simulink model "z5234550RundongGuanPrimaryDT1_2020"  (R2020a)
settings: Solver=FixedStepDiscrete  StartTime=0.0  StopTime=1  FixedStep=Ts  RelTol=1e-3
InitFcn:
  | Ts = 1e-6;
  | Tcs = 100e-6;
  | Freq = 51.2;
undefined symbols (not defined in the file or in its folder): DiscIntNeverNeededParam
libraries: powerlib_meascontrol x2, z5234550RundongGuanLib_DT1_2020 x1, simulink x1
settings Model: Creator=Matthew Priestley  LastModifiedBy=Kevin
settings DataIOCC: SaveOutput=off  SignalLogging=off  DSMLogging=off  SaveTime=off  ReturnWorkspaceOutputs=off

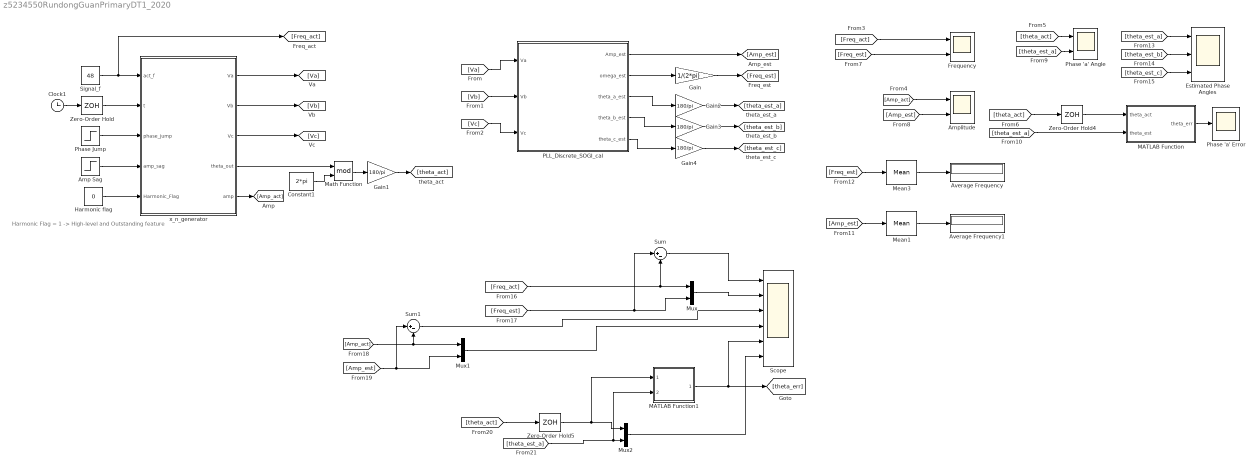
== system z5234550RundongGuanPrimaryDT1_2020 ==
  note: Harmonic Flag = 1 -> High-level and Outstanding feature
  Amp Sag : Step  Before=1  After=0.2  SampleTime=Ts
  Amplitude : Scope  NumInputPorts=2
  Average Frequency : Display
      settings: Decimation=5
  Average Frequency1 : Display
      settings: Decimation=5
  Clock1 : Clock
  Constant1 : Constant  Value=2*pi  SampleTime=Ts  LockScale=on
  Estimated Phase Angles : Scope  NumInputPorts=3
  Frequency : Scope  NumInputPorts=2
  Gain : Gain  Gain=1/(2*pi)
  Gain{1..4} (4 alike) : Gain  Gain=180/pi
  Harmonic flag : Constant  Value=0  SampleTime=Ts  LockScale=on
  MATLAB Function : MATLAB Function  TreatAsAtomicUnit=on
  MATLAB Function1 : MATLAB Function  TreatAsAtomicUnit=on
  Math Function : Math  Operator=mod  SignedPower=on  SaturateOnIntegerOverflow=on
  Mean1 : powerlib_meascontrol/Measurements/Mean  Freq=Freq  Vinit=0  Ts=Ts
  Mean3 : powerlib_meascontrol/Measurements/Mean  Freq=Freq  Vinit=0  Ts=Ts
  Mux : Mux  Inputs=2
  Mux1 : Mux  Inputs=2
  Mux2 : Mux  Inputs=2
  PLL_Discrete_SOGI_cal : Subsystem
  Phase 'a' Angle : Scope  NumInputPorts=2
  Phase 'a' Error : Scope
  Phase Jump : Step  Time=0.5  After=15  SampleTime=Ts
  Scope : Scope  NumInputPorts=6
  Signal_f : Constant  Value=48  SampleTime=Ts  LockScale=on
  Sum : Sum  Inputs=|+-
  Sum1 : Sum  Inputs=|+-
  Zero-Order Hold : ZeroOrderHold  SampleTime=Ts
  Zero-Order Hold4 : ZeroOrderHold  SampleTime=Tcs
  Zero-Order Hold5 : ZeroOrderHold  SampleTime=-1
  x_n_generator : MATLAB Function  TreatAsAtomicUnit=on
  wires:
  x_n_generator/4(theta_out) -> Math Function/1
  Zero-Order Hold/1 -> x_n_generator/2(t)
  x_n_generator/5(amp) -> [Amp_act]
  Phase Jump/1 -> x_n_generator/3(phase_jump)
  Amp Sag/1 -> x_n_generator/4(amp_sag)
  Clock1/1 -> Zero-Order Hold/1
  Math Function/1 -> Gain1/1
  Constant1/1 -> Math Function/2
  x_n_generator/2(Vb) -> [Vb]
  x_n_generator/1(Va) -> [Va]
  x_n_generator/3(Vc) -> [Vc]
  Harmonic flag/1 -> x_n_generator/5(Harmonic_Flag)
  [Freq_act] -> Frequency/1
  [Amp_act] -> Amplitude/1
  [theta_act] -> Phase 'a' Angle/1
  [theta_act] -> Zero-Order Hold4/1
  [Freq_est] -> Frequency/2
  [Amp_est] -> Amplitude/2
  [theta_est_a] -> Phase 'a' Angle/2
  MATLAB Function/1(theta_err) -> Phase 'a' Error/1
  [theta_est_a] -> MATLAB Function/2(theta_est)
  [Freq_est] -> Mean3/1
  Mean3/1 -> Average Frequency/1
  Gain1/1 -> [theta_act]
  [theta_est_a] -> Estimated Phase Angles/1
  [theta_est_b] -> Estimated Phase Angles/2
  [theta_est_c] -> Estimated Phase Angles/3
  Mux/1 -> Scope/2
  [Freq_act] -> Mux/1, Sum/2
  [Freq_est] -> Mux/2, Sum/1
  [Amp_act] -> Sum1/2, Mux1/1
  [Amp_est] -> Sum1/1, Mux1/2
  Mux1/1 -> Scope/4
  [theta_est_a] -> MATLAB Function1/2(theta_est), Mux2/2
  Mux2/1 -> Scope/6
  Zero-Order Hold4/1 -> MATLAB Function/1(theta_act)
  [theta_act] -> Zero-Order Hold5/1
  Zero-Order Hold5/1 -> Mux2/1, MATLAB Function1/1(theta_act)
  Gain/1 -> [Freq_est]
  Gain2/1 -> [theta_est_a]
  Gain3/1 -> [theta_est_b]
  Gain4/1 -> [theta_est_c]
  Sum/1 -> Scope/1
  Sum1/1 -> Scope/3
  MATLAB Function1/1(theta_err) -> [theta_err], Scope/5
  [Va] -> PLL_Discrete_SOGI_cal/1(Va)
  [Vb] -> PLL_Discrete_SOGI_cal/2(Vb)
  [Vc] -> PLL_Discrete_SOGI_cal/3(Vc)
  PLL_Discrete_SOGI_cal/2(omega_est) -> Gain/1
  PLL_Discrete_SOGI_cal/3(theta_a_est) -> Gain2/1
  PLL_Discrete_SOGI_cal/4(theta_b_est) -> Gain3/1
  PLL_Discrete_SOGI_cal/5(theta_c_est) -> Gain4/1
  PLL_Discrete_SOGI_cal/1(Amp_est) -> [Amp_est]
  Signal_f/1 -> [Freq_act], x_n_generator/1(act_f)
  Mean1/1 -> Average Frequency1/1
  [Amp_est] -> Mean1/1

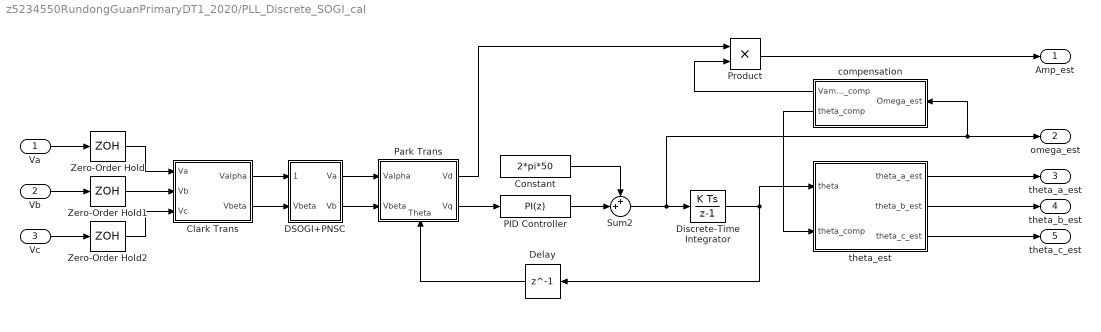
== system z5234550RundongGuanPrimaryDT1_2020/PLL_Discrete_SOGI_cal ==
  Va : Inport
  Vb : Inport  Port=2
  Vc : Inport  Port=3
  Clark Trans : Subsystem
  Constant : Constant  Value=2*pi*50  SampleTime=Tcs
  DSOGI+PNSC : Subsystem
  Delay : Delay  DelayLength=1  SampleTime=Tcs
  Discrete-Time Integrator : DiscreteIntegrator  SampleTime=Tcs  ICPrevOutput=DiscIntNeverNeededParam  ICPrevScaledInput=DiscIntNeverNeededParam
  PID Controller : simulink/Continuous/PID Controller  Controller=PI  Form=Parallel  TimeDomain=Discrete-time  UseExternalTs=off  SampleTime=Tcs  IntegratorMethod=Forward Euler  FilterMethod=Forward Euler  ControllerParametersSource=internal  P=4  I=100  D=0  UseFilter=on  N=100  TunerSelectOption=Transfer Function Based (PID Tuner App)  InitialConditionSource=internal  InitialConditionForIntegrator=0  InitialConditionForFilter=0  DifferentiatorICPrevScaledInput=0  ExternalReset=none  TrackingMode=off  Kt=1  LimitOutput=off  UpperSaturationLimit=inf  LowerSaturationLimit=-inf  LinearizeAsGain=on  AntiWindupMode=none  Kb=1  POutMin=[]  POutMax=[]  IOutMin=[]  IOutMax=[]  DOutMin=[]  DOutMax=[]  NOutMin=[]  NOutMax=[]  SumOutMin=[]  SumOutMax=[]  SaturationOutMin=[]  SaturationOutMax=[]  PParamMin=[]  PParamMax=[]  IParamMin=[]  IParamMax=[]  DParamMin=[]  DParamMax=[]  NParamMin=[]  NParamMax=[]  KbParamMin=[]  KbParamMax=[]  KtParamMin=[]  KtParamMax=[]  KbOutMin=[]  KbOutMax=[]  KtOutMin=[]  KtOutMax=[]  IntegratorOutMin=[]  IntegratorOutMax=[]  FilterOutMin=[]  FilterOutMax=[]  SumI1OutMin=[]  SumI1OutMax=[]  SumI2OutMin=[]  SumI2OutMax=[]  SumI3OutMin=[]  SumI3OutMax=[]  SumI4OutMin=[]  SumI4OutMax=[]  SumDOutMin=[]  SumDOutMax=[]  DifferentiatorOutMin=[]  DifferentiatorOutMax=[]  FilterDiffOutCoefMin=[]  FilterDiffOutCoefMax=[]  ReciprocalOutMin=[]  ReciprocalOutMax=[]  SumDenOutMin=[]  SumDenOutMax=[]  SumNumOutMin=[]  SumNumOutMax=[]  DivideOutMin=[]  DivideOutMax=[]  UdiffTsProdOutMin=[]  UdiffTsProdOutMax=[]  NTsProdOutMin=[]  NTsProdOutMax=[]  UintegralTsProdOutMin=[]  UintegralTsProdOutMax=[]  UngainTsProdOutMin=[]  UngainTsProdOutMax=[]  IntegratorContinuousStateAttributes=''  IntegratorStateMustResolveToSignalObject=off  IntegratorRTWStateStorageClass=Auto  FilterContinuousStateAttributes=''  FilterStateMustResolveToSignalObject=off  FilterRTWStateStorageClass=Auto  ParallelPVariant=InternalParameters  IdealPVariant=Disabled  IVariant=InternalParameters  DVariant=Disabled  IntegratorVariant=Discrete  SatVariant=Disabled  AWVariant=Passthrough  PCopyVariant=Disabled  TRVariant=Disabled  FdbkBlocksVariant=Forward  IdealPFdbkVariant=Disabled  SatFdbkVariant=Disabled  DerivativeFilterVariant=Disabled  NVariant=Disabled  NCopyVariant=Disabled_SignalSpec  FilterICVariant=Disabled  IntegratorICVariant=InternalICs  ExternalResetVariant=Disabled  TRSumVariant=Passthrough  SumFdbkVariant=Disabled  SumVariant=Sum_PI  TsampFilterVariant=InternalTs  TsampNgainVariant=Passthrough  TsampIntegralVariant=Passthrough
  Park Trans : Subsystem
      settings: PortSchema="{\"entries\":[{\"content\":{\"sides\":[{\"content\":{\"connectorIds\":[\"In1\",\"In2\"]},\"type\":\"ConnectorPlacement.EquallySpacedRectSide\",\"uuid\":\"d7ee73cc-3741-4077-b32c-689f2c701f83\"},{\"content\":{\"connectorIds\":[\"Out1\",\"Out2\"],\"side\":\"RIGHT\"},\"type\":\"ConnectorPlacement.EquallySpacedRectSide\",\"uuid\":\"fa84044a-ecd8-49d8-a4b2-ae549d89fe8f\"},{\"content\":{\"connectorIds\":[],\"side\":\"TOP\"},\"type\":\"ConnectorPlacement.EquallySpacedRectSide\",\"uuid\":\"692e7773-1833-4597-a5fd-7846ecf4550e\"},{\"content\":{\"connectorIds\":[\"In3\"],\"side\":\"BOTTOM\"},\"type\":\"ConnectorPlacement.EquallySpacedRectSide\",\"uuid\":\"73d654b9-9f56-4244-9824-eb13bf44a38f\"}]},\"type\":\"ConnectorPlacement.EquallySpacedConnector\",\"uuid\":\"4e0b4972-389e-416e-b0d9-9fdc8ba0f1f7\"}],\"packageUris\":[\"http://schema.mathworks.com/mf0/Connector/19700101\"],\"version\":\"1.0\"}"
  Product : Product
  Sum2 : Sum  Inputs=++|
  Zero-Order Hold : ZeroOrderHold  SampleTime=Tcs
  Zero-Order Hold1 : ZeroOrderHold  SampleTime=Tcs
  Zero-Order Hold2 : ZeroOrderHold  SampleTime=Tcs
  compensation : Subsystem
      settings: PortSchema="{\"entries\":[{\"content\":{\"sides\":[{\"content\":{\"connectorIds\":[\"Out1\",\"Out2\"]},\"type\":\"ConnectorPlacement.EquallySpacedRectSide\",\"uuid\":\"1da655cf-4ef1-485d-9c9d-29e08b49196c\"},{\"content\":{\"connectorIds\":[\"In1\"],\"side\":\"RIGHT\"},\"type\":\"ConnectorPlacement.EquallySpacedRectSide\",\"uuid\":\"274b50d4-d2b9-4d73-9fa7-29da8dc32335\"},{\"content\":{\"connectorIds\":[],\"side\":\"TOP\"},\"type\":\"ConnectorPlacement.EquallySpacedRectSide\",\"uuid\":\"51928977-61f6-4419-af9c-6bbf4ccbe560\"}]},\"type\":\"ConnectorPlacement.EquallySpacedConnector\",\"uuid\":\"bbbb2fbe-31dd-41e3-8294-b416b392d210\"}],\"packageUris\":[\"http://schema.mathworks.com/mf0/Connector/19700101\"],\"version\":\"1.0\"}"
  theta_est : Subsystem
  Amp_est : Outport
  omega_est : Outport  Port=2
  theta_a_est : Outport  Port=3
  theta_b_est : Outport  Port=4
  theta_c_est : Outport  Port=5
  wires:
  compensation/2(theta_comp) -> theta_est/2(theta_comp)
  Park Trans/1(Vd) -> Product/1
  compensation/1(Vamp_comp) -> Product/2
  Product/1 -> Amp_est/1
  Sum2/1 -> Discrete-Time Integrator/1, omega_est/1, compensation/1(Omega_est)
  Zero-Order Hold1/1 -> Clark Trans/2(Vb)
  Vc/1 -> Zero-Order Hold2/1
  Vb/1 -> Zero-Order Hold1/1
  Zero-Order Hold2/1 -> Clark Trans/3(Vc)
  Zero-Order Hold/1 -> Clark Trans/1(Va)
  Va/1 -> Zero-Order Hold/1
  theta_est/1(theta_a_est) -> theta_a_est/1
  theta_est/2(theta_b_est) -> theta_b_est/1
  theta_est/3(theta_c_est) -> theta_c_est/1
  Park Trans/2(Vq) -> PID Controller/1
  Clark Trans/1(Valpha) -> DSOGI+PNSC/1(Valpha)
  Clark Trans/2(Vbeta) -> DSOGI+PNSC/2(Vbeta)
  DSOGI+PNSC/1(Va) -> Park Trans/1(Valpha)
  DSOGI+PNSC/2(Vb) -> Park Trans/2(Vbeta)
  Delay/1 -> Park Trans/3(Theta)
  PID Controller/1 -> Sum2/2
  Constant/1 -> Sum2/1
  Discrete-Time Integrator/1 -> theta_est/1(theta), Delay/1

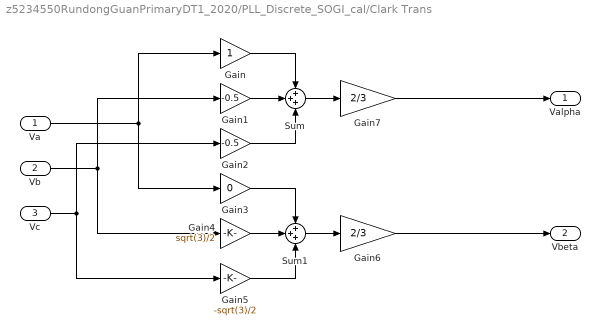
== system z5234550RundongGuanPrimaryDT1_2020/PLL_Discrete_SOGI_cal/Clark Trans ==
  Va : Inport
  Vb : Inport  Port=2
  Vc : Inport  Port=3
  Gain : Gain
  Gain1 : Gain  Gain=-0.5
  Gain2 : Gain  Gain=-0.5
  Gain3 : Gain  Gain=0
  Gain4 : Gain  Gain=sqrt(3)/2
  Gain5 : Gain  Gain=-sqrt(3)/2
  Gain6 : Gain  Gain=2/3
  Gain7 : Gain  Gain=2/3
  Sum : Sum  Inputs=+++
  Sum1 : Sum  Inputs=+++
  Valpha : Outport
  Vbeta : Outport  Port=2
  wires:
  Gain2/1 -> Sum/3
  Va/1 -> Gain3/1, Gain/1
  Vc/1 -> Gain5/1, Gain2/1
  Vb/1 -> Gain4/1, Gain1/1
  Gain/1 -> Sum/1
  Gain3/1 -> Sum1/1
  Gain1/1 -> Sum/2
  Gain5/1 -> Sum1/3
  Gain4/1 -> Sum1/2
  Sum/1 -> Gain7/1
  Sum1/1 -> Gain6/1
  Gain7/1 -> Valpha/1
  Gain6/1 -> Vbeta/1

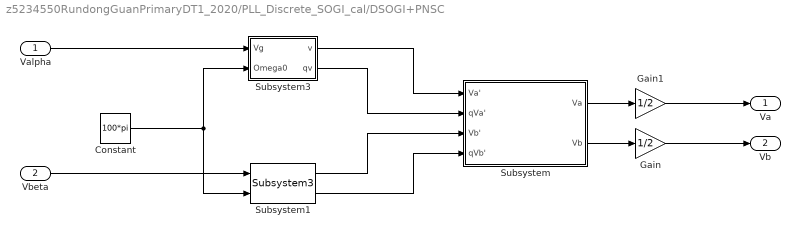
== system z5234550RundongGuanPrimaryDT1_2020/PLL_Discrete_SOGI_cal/DSOGI+PNSC ==
  Valpha : Inport
  Vbeta : Inport  Port=2
  Constant : Constant  Value=100*pi
  Gain : Gain  Gain=1/2
  Gain1 : Gain  Gain=1/2
  Subsystem : Subsystem
  Subsystem1 : z5234550RundongGuanLib_DT1_2020/PLL_Discrete_SOGI/DSOGI+PNSC/Subsystem3  SystemSampleTime=-1  Latency=0  AutoFrameSizeCalculation=off
      link override Gain: Gain=0.75
  Subsystem3 : Subsystem
  Va : Outport
  Vb : Outport  Port=2
  wires:
  Constant/1 -> Subsystem1/2, Subsystem3/2(Omega0)
  Subsystem3/1(v) -> Subsystem/1(Va')
  Subsystem3/2(qv) -> Subsystem/2(qVa')
  Subsystem/1(Va) -> Gain1/1
  Subsystem/2(Vb) -> Gain/1
  Valpha/1 -> Subsystem3/1(Vg)
  Vbeta/1 -> Subsystem1/1
  Subsystem1/1 -> Subsystem/3(Vb')
  Subsystem1/2 -> Subsystem/4(qVb')
  Gain1/1 -> Va/1
  Gain/1 -> Vb/1

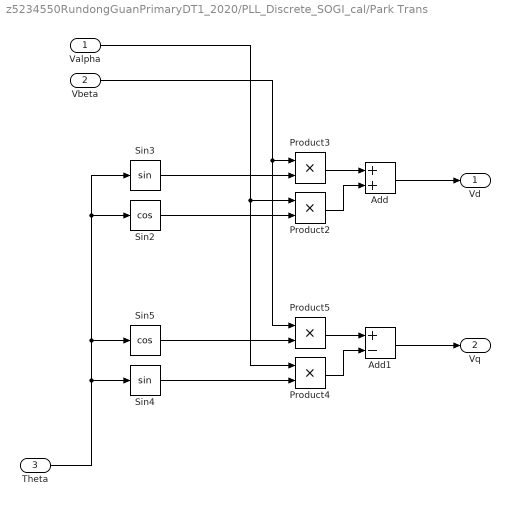
== system z5234550RundongGuanPrimaryDT1_2020/PLL_Discrete_SOGI_cal/Park Trans ==
  Valpha : Inport
  Vbeta : Inport  Port=2
  Theta : Inport  Port=3
  Add : Sum
  Add1 : Sum  Inputs=+-
  Product{2..5} (4 alike) : Product
  Sin2 : Trigonometry  Operator=cos
  Sin3 : Trigonometry
  Sin4 : Trigonometry
  Sin5 : Trigonometry  Operator=cos
  Vd : Outport
  Vq : Outport  Port=2
  wires:
  Vbeta/1 -> Product5/1, Product3/1
  Theta/1 -> Sin4/1, Sin5/1, Sin2/1, Sin3/1
  Sin5/1 -> Product5/2
  Valpha/1 -> Product2/1, Product4/1
  Product4/1 -> Add1/2
  Product2/1 -> Add/2
  Sin2/1 -> Product2/2
  Add/1 -> Vd/1
  Sin3/1 -> Product3/2
  Product3/1 -> Add/1
  Add1/1 -> Vq/1
  Sin4/1 -> Product4/2
  Product5/1 -> Add1/1

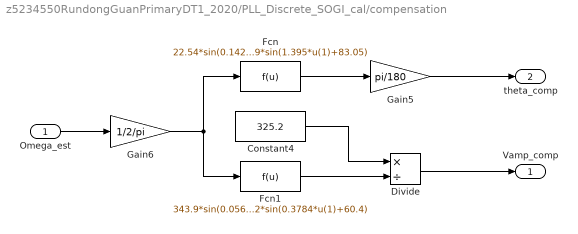
== system z5234550RundongGuanPrimaryDT1_2020/PLL_Discrete_SOGI_cal/compensation ==
  Omega_est : Inport
  Constant4 : Constant  Value=325.2
  Divide : Product  Inputs=*/
  Fcn : Fcn  Expr=22.54*sin(0.1425*u(1)+68.25)+0.07009*sin(1.395*u(1)+83.05)
  Fcn1 : Fcn  Expr=343.9*sin(0.05621*u(1)+36.6)+1.732*sin(0.3784*u(1)+60.4)
  Gain5 : Gain  Gain=pi/180
  Gain6 : Gain  Gain=1/2/pi
  Vamp_comp : Outport
  theta_comp : Outport  Port=2
  wires:
  Gain6/1 -> Fcn/1, Fcn1/1
  Omega_est/1 -> Gain6/1
  Divide/1 -> Vamp_comp/1
  Gain5/1 -> theta_comp/1
  Fcn/1 -> Gain5/1
  Constant4/1 -> Divide/1
  Fcn1/1 -> Divide/2

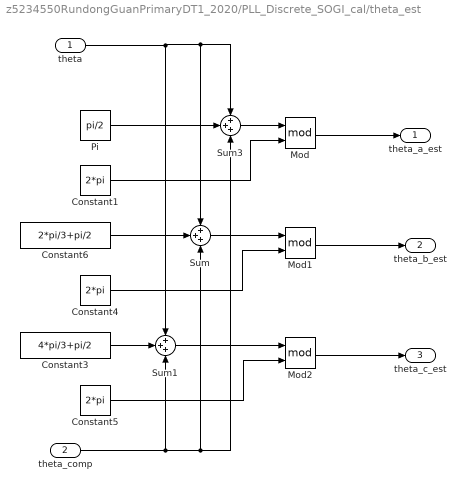
== system z5234550RundongGuanPrimaryDT1_2020/PLL_Discrete_SOGI_cal/theta_est ==
  theta : Inport
  theta_comp : Inport  Port=2
  Constant1 : Constant  Value=2*pi
  Constant3 : Constant  Value=4*pi/3+pi/2
  Constant4 : Constant  Value=2*pi
  Constant5 : Constant  Value=2*pi
  Constant6 : Constant  Value=2*pi/3+pi/2
  Mod : Math  Operator=mod  SaturateOnIntegerOverflow=on
  Mod1 : Math  Operator=mod  SaturateOnIntegerOverflow=on
  Mod2 : Math  Operator=mod  SaturateOnIntegerOverflow=on
  Pi : Constant  Value=pi/2  OutDataTypeStr=Inherit: Inherit via back propagation
  Sum : Sum  Inputs=+++
  Sum1 : Sum  Inputs=+++
  Sum3 : Sum  Inputs=+++
  theta_a_est : Outport
  theta_b_est : Outport  Port=2
  theta_c_est : Outport  Port=3
  wires:
  Mod2/1 -> theta_c_est/1
  Mod1/1 -> theta_b_est/1
  Sum1/1 -> Mod2/1
  Constant4/1 -> Mod1/2
  theta/1 -> Sum1/1, Sum3/1, Sum/1
  Mod/1 -> theta_a_est/1
  Constant6/1 -> Sum/2
  Constant3/1 -> Sum1/2
  Sum3/1 -> Mod/1
  Sum/1 -> Mod1/1
  Constant5/1 -> Mod2/2
  Constant1/1 -> Mod/2
  Pi/1 -> Sum3/2
  theta_comp/1 -> Sum1/3, Sum/3, Sum3/3

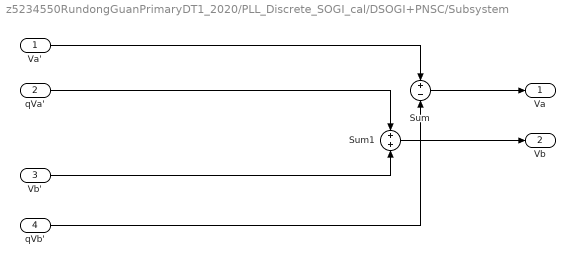
== system z5234550RundongGuanPrimaryDT1_2020/PLL_Discrete_SOGI_cal/DSOGI+PNSC/Subsystem ==
  Va' : Inport
  qVa' : Inport  Port=2
  Vb' : Inport  Port=3
  qVb' : Inport  Port=4
  Sum : Sum  Inputs=+|-
  Sum1 : Sum  Inputs=+|+
  Va : Outport
  Vb : Outport  Port=2
  wires:
  Sum1/1 -> Vb/1
  Sum/1 -> Va/1
  Va'/1 -> Sum/1
  Vb'/1 -> Sum1/2
  qVa'/1 -> Sum1/1
  qVb'/1 -> Sum/2

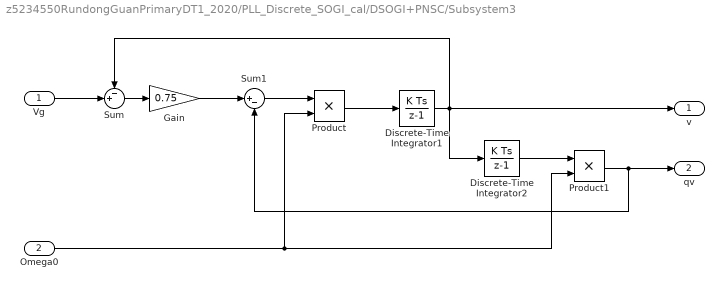
== system z5234550RundongGuanPrimaryDT1_2020/PLL_Discrete_SOGI_cal/DSOGI+PNSC/Subsystem3 ==
  Vg : Inport
  Omega0 : Inport  Port=2
  Discrete-Time Integrator1 : DiscreteIntegrator  SampleTime=Tcs  ICPrevOutput=DiscIntNeverNeededParam  ICPrevScaledInput=DiscIntNeverNeededParam
  Discrete-Time Integrator2 : DiscreteIntegrator  SampleTime=Tcs  ICPrevOutput=DiscIntNeverNeededParam  ICPrevScaledInput=DiscIntNeverNeededParam
  Gain : Gain  Gain=0.75
  Product : Product
  Product1 : Product
  Sum : Sum  Inputs=-+|
  Sum1 : Sum  Inputs=|+-
  v : Outport
  qv : Outport  Port=2
  wires:
  Sum/1 -> Gain/1
  Discrete-Time Integrator1/1 -> v/1, Sum/1, Discrete-Time Integrator2/1
  Omega0/1 -> Product1/2, Product/2
  Product/1 -> Discrete-Time Integrator1/1
  Discrete-Time Integrator2/1 -> Product1/1
  Product1/1 -> qv/1, Sum1/2
  Vg/1 -> Sum/2
  Gain/1 -> Sum1/1
  Sum1/1 -> Product/1

== matlab function z5234550RundongGuanPrimaryDT1_2020/MATLAB Function ==
  data: theta_act input; theta_err output; theta_est input
function theta_err = fcn(theta_act,theta_est)
theta_err = theta_act - theta_est;

if abs(theta_err) > 350
    if (theta_act > 350)&&(theta_est<10)
        theta_err = (theta_act-360) - theta_est;
    elseif (theta_act < 10)&&(theta_est > 350)
        theta_err = (theta_act) - (theta_est-360);
    end
end
        
end

== matlab function z5234550RundongGuanPrimaryDT1_2020/MATLAB Function1 ==
  data: theta_act input; theta_err output; theta_est input
function theta_err = fcn(theta_act,theta_est)
theta_err = theta_act - theta_est;

if abs(theta_err) > 300
    if (theta_act > 300)&&(theta_est<60)
        theta_err = (theta_act-360) - theta_est;
    elseif (theta_act < 60)&&(theta_est > 300)
        theta_err = (theta_act) - (theta_est-360);
    end
end
        
end

== matlab function z5234550RundongGuanPrimaryDT1_2020/x_n_generator ==
  data: act_f input; Va output; Vb output; Vc output; t input; theta_out output; amp output; phase_jump input; amp_sag input; Harmonic_Flag input
function [Va,Vb,Vc,theta_out,amp]  = x_n_generator(act_f,t,phase_jump,amp_sag,Harmonic_Flag)

omega = 2*pi*act_f;

theta = omega*t+phase_jump*pi/180;

V1 = 230*sqrt(2);
amp=V1*amp_sag;
phi = 192.4*pi/180;
V3 = 0.51;
phi3 = 101.4*pi/180;
V5 = 2.08;
phi5 = 223.8*pi/180;
V7 = 3;
phi7 = 121.3*pi/180;
V9 = 0.28;
phi9 = -70.4*pi/180;
V11 = 0.55;
phi11 = 201.4*pi/180;
V13 = 0.61;
phi13 = 53.1*pi/180;

Va1 = V1*sin(theta+phi);
Vb1 = V1*sin(theta+phi-2*pi/3);
Vc1 = V1*sin(theta+phi+2*pi/3);
Va3 = V3*sin(3*(theta)+phi3);
Vb3 = V3*sin(3*(theta-2*pi/3)+phi3);
Vc3 = V3*sin(3*(theta+2*pi/3)+phi3);
Va5 = V5*sin(5*(theta)+phi5);
Vb5 = V5*sin(5*(theta-2*pi/3)+phi5);
Vc5 = V5*sin(5*(theta+2*pi/3)+phi5);
Va7 = V7*sin(7*(theta)+phi7);
Vb7 = V7*sin(7*(theta-2*pi/3)+phi7);
Vc7 = V7*sin(7*(theta+2*pi/3)+phi7);
Va9 = V9*sin(9*(theta)+phi9);
Vb9 = V9*sin(9*(theta-2*pi/3)+phi9);
Vc9 = V9*sin(9*(theta+2*pi/3)+phi9);
Va11 = V11*sin(11*(theta)+phi11);
Vb11 = V11*sin(11*(theta-2*pi/3)+phi11);
Vc11 = V11*sin(11*(theta+2*pi/3)+phi11);
Va13 = V13*sin(13*(theta)+phi13);
Vb13 = V13*sin(13*(theta-2*pi/3)+phi13);
Vc13 = V13*sin(13*(theta+2*pi/3)+phi13);

if Harmonic_Flag == 1
    Va = amp_sag*(Va1+Va3+Va5+Va7+Va9+Va11+Va13);
    Vb = amp_sag*(Vb1+Vb3+Vb5+Vb7+Vb9+Vb11+Vb13);
    Vc = amp_sag*(Vc1+Vc3+Vc5+Vc7+Vc9+Vc11+Vc13);
else
    Va = amp_sag*Va1;
    Vb = amp_sag*Vb1;
    Vc = amp_sag*Vc1;
end

theta_out = theta+phi;

end
